simulink model "part19"  (R2020a)
settings: Solver=VariableStepAuto  StartTime=0.0  StopTime=40.0  RelTol=1e-3
settings Model: Creator=emami  LastModifiedBy=emami

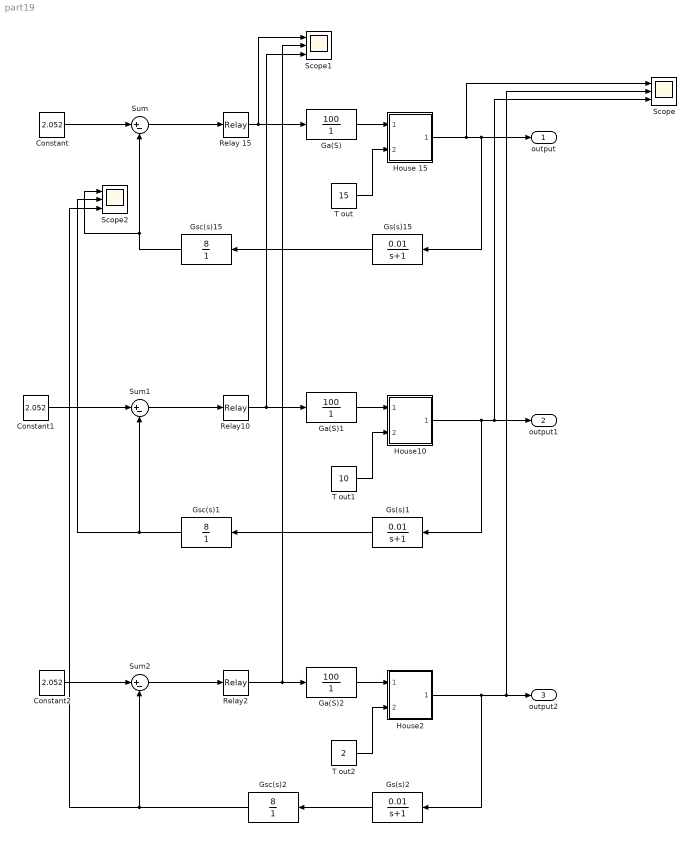
== system part19 ==
  " Gs(s)1" : TransferFcn  Numerator=[0.01]  Denominator=[1 1]
  " Gs(s)15" : TransferFcn  Numerator=[0.01]  Denominator=[1 1]
  " Gs(s)2" : TransferFcn  Numerator=[0.01]  Denominator=[1 1]
  " Gsc(s)1" : TransferFcn  Numerator=[8]  Denominator=[1]
  " Gsc(s)15" : TransferFcn  Numerator=[8]  Denominator=[1]
  " Gsc(s)2" : TransferFcn  Numerator=[8]  Denominator=[1]
  Constant : Constant  Value=2.052
  Constant1 : Constant  Value=2.052
  Constant2 : Constant  Value=2.052
  Ga(S) : TransferFcn  Numerator=[100]  Denominator=[1]
  Ga(S)1 : TransferFcn  Numerator=[100]  Denominator=[1]
  Ga(S)2 : TransferFcn  Numerator=[100]  Denominator=[1]
  House 15 : Subsystem
      mask Display: image(fullfile(matlabroot,'toolbox','simulink','simdemos','simgeneral','images','HouseHeatHousePix.svg'))
  House10 : Subsystem
      mask Display: image(fullfile(matlabroot,'toolbox','simulink','simdemos','simgeneral','images','HouseHeatHousePix.svg'))
  House2 : Subsystem
      mask Display: image(fullfile(matlabroot,'toolbox','simulink','simdemos','simgeneral','images','HouseHeatHousePix.svg'))
  Relay 15 : Relay  OnSwitchValue=0.001  OffSwitchValue=-0.001  OnOutputValue=10
  Relay10 : Relay  OnSwitchValue=0.001  OffSwitchValue=-0.001  OnOutputValue=10
  Relay2 : Relay  OnSwitchValue=0.001  OffSwitchValue=-0.001  OnOutputValue=10
  Scope : Scope  NumInputPorts=3
  Scope1 : Scope  NumInputPorts=3
  Scope2 : Scope  NumInputPorts=3
  Sum : Sum  Inputs=|+-
  Sum1 : Sum  Inputs=|+-
  Sum2 : Sum  Inputs=|+-
  T out : Constant  Value=15
  T out1 : Constant  Value=10
  T out2 : Constant  Value=2
  output : Outport
  output1 : Outport  Port=2
  output2 : Outport  Port=3
  wires:
  Relay 15/1 -> Ga(S)/1, Scope1/1
  Sum/1 -> Relay 15/1
  Constant/1 -> Sum/1
  T out/1 -> House 15/2(Outdoor Temp Tout)
  " Gsc(s)15"/1 -> Scope2/1, Sum/2
  Ga(S)/1 -> House 15/1(Heater QDot In)
  House 15/1(Room Temp Troom) -> Scope/1, " Gs(s)15"/1, output/1
  " Gs(s)15"/1 -> " Gsc(s)15"/1
  Relay10/1 -> Scope1/3, Ga(S)1/1
  Sum1/1 -> Relay10/1
  Constant1/1 -> Sum1/1
  T out1/1 -> House10/2(Outdoor Temp Tout)
  " Gsc(s)1"/1 -> Scope2/2, Sum1/2
  Ga(S)1/1 -> House10/1(Heater QDot In)
  House10/1(Room Temp Troom) -> " Gs(s)1"/1, Scope/3, output1/1
  " Gs(s)1"/1 -> " Gsc(s)1"/1
  Relay2/1 -> Scope1/2, Ga(S)2/1
  Sum2/1 -> Relay2/1
  Constant2/1 -> Sum2/1
  T out2/1 -> House2/2(Outdoor Temp Tout)
  " Gsc(s)2"/1 -> Scope2/3, Sum2/2
  Ga(S)2/1 -> House2/1(Heater QDot In)
  House2/1(Room Temp Troom) -> " Gs(s)2"/1, Scope/2, output2/1
  " Gs(s)2"/1 -> " Gsc(s)2"/1

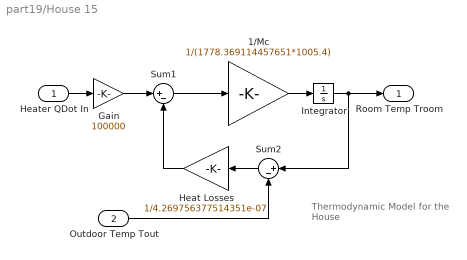
== system part19/House 15 ==
  note: Thermodynamic Model
      | for the House
  Heater QDot In : Inport
  Outdoor Temp Tout : Inport  Port=2
  1/Mc : Gain  Gain=1/(1778.369114457651*1005.4)  SaturateOnIntegerOverflow=on  OutDataTypeStr=Inherit: Same as input  ParamDataTypeStr=Inherit: Same as input
  Gain : Gain  Gain=100000
  Heat Losses : Gain  Gain=1/4.269756377514351e-07  SaturateOnIntegerOverflow=on  OutDataTypeStr=Inherit: Same as input  ParamDataTypeStr=Inherit: Same as input
  Integrator : Integrator  InitialCondition=20
  Sum1 : Sum  Inputs=|+-  InputSameDT=on  SaturateOnIntegerOverflow=on  OutDataTypeStr=Inherit: Same as first input
  Sum2 : Sum  Inputs=|+-  InputSameDT=on  SaturateOnIntegerOverflow=on  OutDataTypeStr=Inherit: Same as first input
  Room Temp Troom : Outport  InitialOutput=0
  wires:
  Outdoor Temp Tout/1 -> Sum2/2
  Heater QDot In/1 -> Gain/1
  Sum1/1 -> 1/Mc/1
  Sum2/1 -> Heat Losses/1
  Heat Losses/1 -> Sum1/2
  1/Mc/1 -> Integrator/1
  Integrator/1 -> Sum2/1, Room Temp Troom/1
  Gain/1 -> Sum1/1

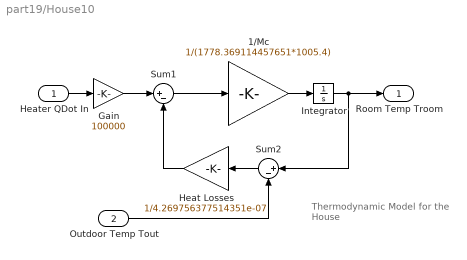
== system part19/House10 ==
  note: Thermodynamic Model
      | for the House
  Heater QDot In : Inport
  Outdoor Temp Tout : Inport  Port=2
  1/Mc : Gain  Gain=1/(1778.369114457651*1005.4)  SaturateOnIntegerOverflow=on  OutDataTypeStr=Inherit: Same as input  ParamDataTypeStr=Inherit: Same as input
  Gain : Gain  Gain=100000
  Heat Losses : Gain  Gain=1/4.269756377514351e-07  SaturateOnIntegerOverflow=on  OutDataTypeStr=Inherit: Same as input  ParamDataTypeStr=Inherit: Same as input
  Integrator : Integrator  InitialCondition=20
  Sum1 : Sum  Inputs=|+-  InputSameDT=on  SaturateOnIntegerOverflow=on  OutDataTypeStr=Inherit: Same as first input
  Sum2 : Sum  Inputs=|+-  InputSameDT=on  SaturateOnIntegerOverflow=on  OutDataTypeStr=Inherit: Same as first input
  Room Temp Troom : Outport  InitialOutput=0
  wires:
  Outdoor Temp Tout/1 -> Sum2/2
  Heater QDot In/1 -> Gain/1
  Sum1/1 -> 1/Mc/1
  Sum2/1 -> Heat Losses/1
  Heat Losses/1 -> Sum1/2
  1/Mc/1 -> Integrator/1
  Integrator/1 -> Sum2/1, Room Temp Troom/1
  Gain/1 -> Sum1/1

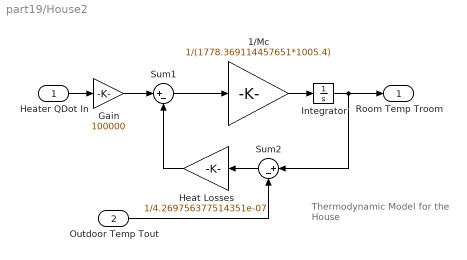
== system part19/House2 ==
  note: Thermodynamic Model
      | for the House
  Heater QDot In : Inport
  Outdoor Temp Tout : Inport  Port=2
  1/Mc : Gain  Gain=1/(1778.369114457651*1005.4)  SaturateOnIntegerOverflow=on  OutDataTypeStr=Inherit: Same as input  ParamDataTypeStr=Inherit: Same as input
  Gain : Gain  Gain=100000
  Heat Losses : Gain  Gain=1/4.269756377514351e-07  SaturateOnIntegerOverflow=on  OutDataTypeStr=Inherit: Same as input  ParamDataTypeStr=Inherit: Same as input
  Integrator : Integrator  InitialCondition=20
  Sum1 : Sum  Inputs=|+-  InputSameDT=on  SaturateOnIntegerOverflow=on  OutDataTypeStr=Inherit: Same as first input
  Sum2 : Sum  Inputs=|+-  InputSameDT=on  SaturateOnIntegerOverflow=on  OutDataTypeStr=Inherit: Same as first input
  Room Temp Troom : Outport  InitialOutput=0
  wires:
  Outdoor Temp Tout/1 -> Sum2/2
  Heater QDot In/1 -> Gain/1
  Sum1/1 -> 1/Mc/1
  Sum2/1 -> Heat Losses/1
  Heat Losses/1 -> Sum1/2
  1/Mc/1 -> Integrator/1
  Integrator/1 -> Sum2/1, Room Temp Troom/1
  Gain/1 -> Sum1/1
